simulink model "DLHnguoc_5DOF"  (R2018a)
settings: Solver=VariableStepAuto  StartTime=0.0  StopTime=10.0  RelTol=1e-3
settings Model: Creator=Dell  LastModifiedBy=Nguyen Mai

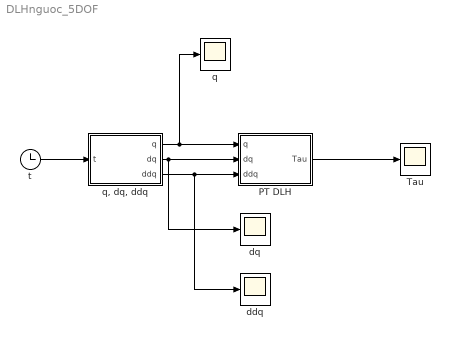
== system DLHnguoc_5DOF ==
  PT DLH : MATLAB Function  TreatAsAtomicUnit=on
  Tau : Scope
  ddq : Scope
  dq : Scope
  q : Scope
  "q, dq, ddq" : MATLAB Function  TreatAsAtomicUnit=on
  t : Clock
  wires:
  "q, dq, ddq"/1(q) -> q/1, PT DLH/1(q)
  t/1 -> "q, dq, ddq"/1(t)
  "q, dq, ddq"/2(dq) -> dq/1, PT DLH/2(dq)
  "q, dq, ddq"/3(ddq) -> ddq/1, PT DLH/3(ddq)
  PT DLH/1(Tau) -> Tau/1

== matlab function DLHnguoc_5DOF/PT DLH ==
  data: q input; Tau output; dq input; ddq input
function Tau=DLHN(q,dq,ddq)
[m1,m2,m3,m4,m5,L1,L2,L3,L4,L5,Lc1,Lc2,Lc3,Lc4,Lc5,g,I1x,I1y,I1z,I2x,I2y,I2z,I3x,I3y,I3z,I4x,I4y,I4z,I5x,I5y,I5z]=parameter ();
ddq=zeros(5,1);
% Khai bao ma tran khoi luong M
M=zeros(5,5);
M(1,1)= m4*L3^2*cos(q(3))^2+m4*cos(q(3))^2*L4^2+I3z+I2y+I1z+(9/4)*m3*L3^2*cos(q(3))^2-(9/4)*L5^2*cos(q(5))^2*cos(q(4))^2*cos(q(3))^2*m5+(9/4)*m2*L2^2-3*m5*cos(q(3))*L5*sin(q(5))*L2+cos(q(3))^2*cos(q(4))^2*I4x+m5*L3^2*cos(q(3))^2+m5*cos(q(3))^2*L4^2-I4y*cos(q(3))^2+cos(q(3))^2*I4z+(1/4)*m4*L4^2+m5*L2^2+I5x*cos(q(3))^2*cos(q(5))^2+I5y*cos(q(4))^2*cos(q(3))^2-I5y*cos(q(3))^2*cos(q(5))^2-I5z*cos(q(4))^2*cos(q(3))^2+(9/4)*L5^2*cos(q(5))^2*m5-2*I5x*cos(q(4))*cos(q(3))*sin(q(3))*cos(q(5))*sin(q(5))+2*I5y*cos(q(4))*cos(q(3))*sin(q(3))*cos(q(5))*sin(q(5))+3*L2*L3*cos(q(3))*m3-(1/4)*L4^2*cos(q(4))^2*cos(q(3))^2*m4+cos(q(3))^2*I3x-I3z*cos(q(3))^2-I5x*cos(q(3))^2-I5x*cos(q(5))^2+I5y*cos(q(5))^2+cos(q(3))^2*I5z-m4*L4*cos(q(4))*sin(q(3))*L2-I4z*cos(q(4))^2*cos(q(3))^2+L2^2*m3+(9/4)*m5*cos(q(3))^2*L5^2+2*m4*cos(q(3))^2*L4*L3+m4*L2^2-I5y*cos(q(4))^2*cos(q(3))^2*cos(q(5))^2-(9/4)*L5^2*cos(q(5))^2*cos(q(3))^2*m5+2*m4*L3*cos(q(3))*L2+2*m4*cos(q(3))*L4*L2+I5x-m4*cos(q(3))*L4^2*sin(q(3))*cos(q(4))+I5x*cos(q(4))^2*cos(q(3))^2*cos(q(5))^2+2*m5*L3*cos(q(3))*L2+2*m5*cos(q(3))*L4*L2+I4y-m4*L3*cos(q(3))*sin(q(3))*cos(q(4))*L4-3*m5*L5*cos(q(5))*cos(q(4))*sin(q(3))*L2+(9/2)*m5*sin(q(3))*cos(q(4))*L5^2*cos(q(5))*cos(q(3))*sin(q(5))-3*m5*sin(q(3))*cos(q(4))*L5*cos(q(5))*L3*cos(q(3))-3*m5*sin(q(3))*cos(q(4))*L5*cos(q(5))*cos(q(3))*L4+2*m5*L3*cos(q(3))^2*L4-3*m5*cos(q(3))^2*L5*sin(q(5))*L3-3*m5*cos(q(3))^2*L5*sin(q(5))*L4;
M(1,2)= 0;
M(1,3)= (1/4)*sin(q(4))*(-9*m5*L5^2*cos(q(5))^2*cos(q(4))*cos(q(3))+9*m5*L5^2*sin(q(5))*cos(q(5))*sin(q(3))+4*I5x*cos(q(5))^2*cos(q(4))*cos(q(3))-4*I5y*cos(q(5))^2*cos(q(4))*cos(q(3))-6*m5*L3*L5*cos(q(5))*sin(q(3))-m4*L4^2*cos(q(4))*cos(q(3))-6*m5*L4*L5*cos(q(5))*sin(q(3))-4*I5x*sin(q(5))*cos(q(5))*sin(q(3))+4*I5y*sin(q(5))*cos(q(5))*sin(q(3))-2*m4*L3*L4*sin(q(3))-2*m4*L4^2*sin(q(3))+4*I4x*cos(q(4))*cos(q(3))-4*I4z*cos(q(4))*cos(q(3))+4*I5y*cos(q(4))*cos(q(3))-4*I5z*cos(q(4))*cos(q(3)));
M(1,4)= (1/4)*m4*L4^2*sin(q(3))-(1/2)*m4*L4^2*cos(q(4))*cos(q(3))-(1/2)*m4*L4*L3*cos(q(4))*cos(q(3))-(1/2)*m4*L4*L2*cos(q(4))+I4y*sin(q(3))-I5x*cos(q(5))^2*sin(q(3))+I5y*cos(q(5))^2*sin(q(3))+(9/4)*m5*L5^2*cos(q(5))^2*sin(q(3))+I5y*sin(q(5))*cos(q(5))*cos(q(4))*cos(q(3))+I5x*sin(q(3))-I5x*sin(q(5))*cos(q(5))*cos(q(4))*cos(q(3))-(3/2)*m5*L5*cos(q(5))*L3*cos(q(4))*cos(q(3))-(3/2)*m5*L5*cos(q(5))*L4*cos(q(4))*cos(q(3))+(9/4)*m5*L5^2*cos(q(5))*sin(q(5))*cos(q(4))*cos(q(3))-(3/2)*m5*L5*cos(q(5))*L2*cos(q(4));
M(1,5)= -(1/4)*sin(q(4))*(-6*m5*L5*L3*sin(q(5))*cos(q(3))-6*m5*L5*L4*sin(q(5))*cos(q(3))-6*m5*L5*L2*sin(q(5))+9*m5*L5^2*cos(q(3))+4*I5z*cos(q(3)));

M(2,1)=0;
M(2,2)=(1/4)*m1;
M(2,3)=0;
M(2,4)=0;
M(2,5)=0;

M(3,1)=(1/4)*sin(q(4))*(-9*m5*L5^2*cos(q(5))^2*cos(q(4))*cos(q(3))+9*m5*L5^2*sin(q(5))*cos(q(5))*sin(q(3))+4*I5x*cos(q(5))^2*cos(q(4))*cos(q(3))-4*I5y*cos(q(5))^2*cos(q(4))*cos(q(3))-6*m5*L3*L5*cos(q(5))*sin(q(3))-m4*L4^2*cos(q(4))*cos(q(3))-6*m5*L4*L5*cos(q(5))*sin(q(3))-4*I5x*sin(q(5))*cos(q(5))*sin(q(3))+4*I5y*sin(q(5))*cos(q(5))*sin(q(3))-2*m4*L3*L4*sin(q(3))-2*m4*L4^2*sin(q(3))+4*I4x*cos(q(4))*cos(q(3))-4*I4z*cos(q(4))*cos(q(3))+4*I5y*cos(q(4))*cos(q(3))-4*I5z*cos(q(4))*cos(q(3)));
M(3,2)=0;
M(3,3)=(9/4)*m3*L3^2+I3y+m4*L3^2+I4z*cos(q(4))^2-I4x*cos(q(4))^2+m4*L4^2+2*m4*L4*L3+(1/4)*m4*cos(q(4))^2*L4^2+I4x+I5y*cos(q(4))^2*cos(q(5))^2-I5x*cos(q(4))^2*cos(q(5))^2+(9/4)*m5*cos(q(4))^2*L5^2*cos(q(5))^2+m5*L3^2+m5*L4^2+2*m5*L3*L4-(9/4)*L5^2*cos(q(5))^2*m5+(9/4)*m5*L5^2-3*L4*L5*sin(q(5))*m5-3*L3*L5*sin(q(5))*m5+I5z*cos(q(4))^2+I5x*cos(q(5))^2-I5y*cos(q(4))^2-I5y*cos(q(5))^2+I5y;
M(3,4)=-(1/4)*sin(q(4))*(-9*L5^2*sin(q(5))*cos(q(5))*m5+6*L3*L5*cos(q(5))*m5+6*L4*L5*cos(q(5))*m5+4*I5x*sin(q(5))*cos(q(5))-4*I5y*sin(q(5))*cos(q(5))+2*m4*L4*L3+2*m4*L4^2);
M(3,5)=(1/4)*cos(q(4))*(-6*L3*L5*sin(q(5))*m5-6*L4*L5*sin(q(5))*m5+9*m5*L5^2+4*I5z);

M(4,1)=(1/4)*m4*L4^2*sin(q(3))-(1/2)*m4*L4^2*cos(q(4))*cos(q(3))-(1/2)*m4*L4*L3*cos(q(4))*cos(q(3))-(1/2)*m4*L4*L2*cos(q(4))+I4y*sin(q(3))-I5x*cos(q(5))^2*sin(q(3))+I5y*cos(q(5))^2*sin(q(3))+(9/4)*m5*L5^2*cos(q(5))^2*sin(q(3))+I5y*sin(q(5))*cos(q(5))*cos(q(4))*cos(q(3))+I5x*sin(q(3))-I5x*sin(q(5))*cos(q(5))*cos(q(4))*cos(q(3))-(3/2)*m5*L5*cos(q(5))*L3*cos(q(4))*cos(q(3))-(3/2)*m5*L5*cos(q(5))*L4*cos(q(4))*cos(q(3))+(9/4)*m5*L5^2*cos(q(5))*sin(q(5))*cos(q(4))*cos(q(3))-(3/2)*m5*L5*cos(q(5))*L2*cos(q(4));
M(4,2)=0;
M(4,3)=-(1/4)*sin(q(4))*(-9*L5^2*sin(q(5))*cos(q(5))*m5+6*L3*L5*cos(q(5))*m5+6*L4*L5*cos(q(5))*m5+4*I5x*sin(q(5))*cos(q(5))-4*I5y*sin(q(5))*cos(q(5))+2*m4*L4*L3+2*m4*L4^2);
M(4,4)=(1/4)*m4*L4^2+I4y+I5y*cos(q(5))^2-I5x*cos(q(5))^2+I5x+(9/4)*L5^2*cos(q(5))^2*m5;
M(4,5)=0;

M(5,1)=-(1/4)*sin(q(4))*(-6*m5*L5*L3*sin(q(5))*cos(q(3))-6*m5*L5*L4*sin(q(5))*cos(q(3))-6*m5*L5*L2*sin(q(5))+9*m5*L5^2*cos(q(3))+4*I5z*cos(q(3)));
M(5,2)=0;
M(5,3)=(1/4)*cos(q(4))*(-6*L3*L5*sin(q(5))*m5-6*L4*L5*sin(q(5))*m5+9*m5*L5^2+4*I5z);
M(5,4)=0;
M(5,5)=(9/4)*m5*L5^2+I5z;

% Khai bao ma tran Coriolis C
%h=-m2*L1*Lc2*sin(q(2));
Co=zeros(5,5);
Co(1,1)=-2*sin(q(4))*dq(4)*cos(q(3))^2*cos(q(4))*I4x-2*sin(q(4))*dq(4)*I5y*cos(q(4))*cos(q(3))^2+2*sin(q(4))*dq(4)*I5z*cos(q(4))*cos(q(3))^2+2*sin(q(4))*dq(4)*I4z*cos(q(4))*cos(q(3))^2-2*dq(3)*m4*cos(q(3))^2*L4^2*cos(q(4))-2*dq(3)*m4*sin(q(3))*L4*L2-2*dq(3)*m4*cos(q(3))*L4^2*sin(q(3))-2*dq(3)*m4*L3*sin(q(3))*L2-2*dq(3)*m5*L3*sin(q(3))*L2-2*dq(3)*m5*sin(q(3))*L4*L2-2*dq(3)*m4*L3^2*cos(q(3))*sin(q(3))-(9/2)*dq(3)*m3*L3^2*cos(q(3))*sin(q(3))-2*dq(3)*cos(q(3))*cos(q(4))^2*I4x*sin(q(3))-2*dq(3)*m5*L3^2*cos(q(3))*sin(q(3))-2*dq(3)*m5*cos(q(3))*L4^2*sin(q(3))-2*dq(3)*I5x*cos(q(3))*cos(q(5))^2*sin(q(3))-2*dq(3)*I5y*cos(q(4))^2*cos(q(3))*sin(q(3))+2*dq(3)*I5y*cos(q(3))*cos(q(5))^2*sin(q(3))+2*dq(3)*I5z*cos(q(4))^2*cos(q(3))*sin(q(3))-3*dq(3)*L2*L3*sin(q(3))*m3+2*dq(3)*I4z*cos(q(4))^2*cos(q(3))*sin(q(3))-(9/2)*dq(3)*m5*cos(q(3))*L5^2*sin(q(3))+2*dq(5)*I5x*cos(q(4))*cos(q(3))*sin(q(3))-2*dq(5)*I5y*cos(q(4))*cos(q(3))*sin(q(3))-2*dq(5)*I5x*cos(q(3))^2*cos(q(5))*sin(q(5))+2*dq(5)*I5y*cos(q(3))^2*cos(q(5))*sin(q(5))-(9/2)*L5^2*cos(q(4))*sin(q(5))*cos(q(5))*dq(3)*m5-(9/2)*L5^2*sin(q(5))*cos(q(5))*dq(5)*m5+2*I5x*cos(q(4))*sin(q(5))*cos(q(5))*dq(3)-2*I5y*cos(q(4))*sin(q(5))*cos(q(5))*dq(3)+L3*L4*cos(q(4))*dq(3)*m4+2*dq(3)*I4y*cos(q(3))*sin(q(3))-2*dq(3)*cos(q(3))*I3x*sin(q(3))+2*dq(3)*I3z*cos(q(3))*sin(q(3))+2*dq(3)*I5x*cos(q(3))*sin(q(3))-2*dq(3)*cos(q(3))*I5z*sin(q(3))-2*dq(3)*cos(q(3))*I4z*sin(q(3))+3*sin(q(4))*dq(4)*m5*sin(q(3))*L5*cos(q(5))*cos(q(3))*L4+3*sin(q(4))*dq(4)*m5*sin(q(3))*L5*cos(q(5))*L3*cos(q(3))-(9/2)*sin(q(4))*dq(4)*m5*sin(q(3))*L5^2*cos(q(5))*cos(q(3))*sin(q(5))+3*dq(5)*m5*sin(q(3))*cos(q(4))*L5*sin(q(5))*cos(q(3))*L4+3*dq(5)*m5*sin(q(3))*cos(q(4))*L5*sin(q(5))*L3*cos(q(3))+(9/2)*sin(q(4))*dq(4)*L5^2*cos(q(5))^2*cos(q(4))*cos(q(3))^2*m5+2*sin(q(4))*dq(4)*I5x*cos(q(3))*sin(q(3))*cos(q(5))*sin(q(5))-2*sin(q(4))*dq(4)*I5y*cos(q(3))*sin(q(3))*cos(q(5))*sin(q(5))+sin(q(4))*dq(4)*m4*cos(q(3))*L4*L3*sin(q(3))+3*sin(q(4))*dq(4)*m5*L5*cos(q(5))*sin(q(3))*L2+9*dq(3)*m5*cos(q(3))^2*cos(q(4))*L5^2*cos(q(5))*sin(q(5))-6*dq(3)*m5*cos(q(3))^2*cos(q(4))*L5*cos(q(5))*L3-6*dq(3)*m5*cos(q(3))^2*cos(q(4))*L5*cos(q(5))*L4-3*dq(3)*m5*L5*cos(q(5))*cos(q(4))*cos(q(3))*L2+6*dq(3)*m5*cos(q(3))*L5*sin(q(5))*L3*sin(q(3))+6*dq(3)*m5*cos(q(3))*L5*sin(q(5))*L4*sin(q(3))+(9/2)*dq(3)*L5^2*cos(q(5))^2*cos(q(4))^2*cos(q(3))*m5*sin(q(3))+(9/2)*dq(5)*L5^2*cos(q(5))*cos(q(4))^2*cos(q(3))^2*m5*sin(q(5))+9*dq(5)*m5*sin(q(3))*cos(q(4))*L5^2*cos(q(5))^2*cos(q(3))+3*dq(5)*m5*L5*sin(q(5))*cos(q(4))*sin(q(3))*L2+(1/2)*sin(q(4))*dq(4)*m4*cos(q(3))^2*L4^2*cos(q(4))+sin(q(4))*dq(4)*m4*sin(q(3))*L4*L2+2*sin(q(4))*dq(4)*I5y*cos(q(4))*cos(q(3))^2*cos(q(5))^2+sin(q(4))*dq(4)*m4*cos(q(3))*L4^2*sin(q(3))-2*sin(q(4))*dq(4)*I5x*cos(q(4))*cos(q(3))^2*cos(q(5))^2-4*dq(3)*m4*cos(q(3))*L4*L3*sin(q(3))-2*dq(3)*I5x*cos(q(4))^2*cos(q(3))*cos(q(5))^2*sin(q(3))-4*dq(3)*m5*L3*cos(q(3))*L4*sin(q(3))+3*dq(3)*m5*sin(q(3))*L5*sin(q(5))*L2+(1/2)*dq(3)*L4^2*cos(q(4))^2*cos(q(3))*m4*sin(q(3))-dq(3)*m4*L4*cos(q(4))*cos(q(3))*L2+2*dq(3)*I5y*cos(q(4))^2*cos(q(3))*cos(q(5))^2*sin(q(3))+(9/2)*dq(3)*L5^2*cos(q(5))^2*cos(q(3))*m5*sin(q(3))-2*dq(3)*m4*L3*cos(q(3))^2*cos(q(4))*L4-4*dq(3)*I5x*cos(q(4))*cos(q(3))^2*cos(q(5))*sin(q(5))+4*dq(3)*I5y*cos(q(4))*cos(q(3))^2*cos(q(5))*sin(q(5))-(9/2)*dq(5)*m5*sin(q(3))*cos(q(4))*L5^2*cos(q(3))-2*dq(5)*I5x*cos(q(4))^2*cos(q(3))^2*cos(q(5))*sin(q(5))+2*dq(5)*I5y*cos(q(4))^2*cos(q(3))^2*cos(q(5))*sin(q(5))+(9/2)*dq(5)*L5^2*cos(q(5))*cos(q(3))^2*m5*sin(q(5))-4*dq(5)*I5x*cos(q(4))*cos(q(3))*sin(q(3))*cos(q(5))^2+4*dq(5)*I5y*cos(q(4))*cos(q(3))*sin(q(3))*cos(q(5))^2-3*dq(5)*m5*cos(q(3))^2*L5*cos(q(5))*L3-3*dq(5)*m5*cos(q(3))^2*L5*cos(q(5))*L4-3*dq(5)*m5*cos(q(3))*L5*cos(q(5))*L2+3*L3*L5*cos(q(4))*cos(q(5))*dq(3)*m5+3*L4*L5*cos(q(4))*cos(q(5))*dq(3)*m5+2*I5x*sin(q(5))*cos(q(5))*dq(5)-2*I5y*sin(q(5))*cos(q(5))*dq(5)+L4^2*cos(q(4))*dq(3)*m4;
Co(1,2)=0;
Co(1,3)=-sin(q(4))*dq(3)*I5x*cos(q(5))^2*cos(q(4))*sin(q(3))+sin(q(4))*dq(3)*I5y*cos(q(5))^2*cos(q(4))*sin(q(3))+(1/4)*sin(q(4))*dq(3)*L4^2*cos(q(4))*sin(q(3))*m4-sin(q(4))*dq(3)*I5x*cos(q(5))*cos(q(3))*sin(q(5))+sin(q(4))*dq(3)*I5y*cos(q(5))*cos(q(3))*sin(q(5))-(1/2)*sin(q(4))*dq(3)*m4*L4*L3*cos(q(3))-(9/2)*dq(4)*L5^2*cos(q(4))^2*cos(q(5))^2*cos(q(3))*m5-dq(4)*I5x*cos(q(4))*sin(q(5))*cos(q(5))*sin(q(3))+dq(4)*I5y*cos(q(4))*sin(q(5))*cos(q(5))*sin(q(3))-(1/2)*dq(4)*L3*L4*cos(q(4))*sin(q(3))*m4+(9/2)*L5^2*cos(q(5))^2*sin(q(3))*sin(q(4))*dq(5)*m5-(1/2)*sin(q(4))*dq(3)*m4*L4^2*cos(q(3))-sin(q(4))*dq(3)*I4x*cos(q(4))*sin(q(3))+sin(q(4))*dq(3)*I4z*cos(q(4))*sin(q(3))-sin(q(4))*dq(3)*I5y*cos(q(4))*sin(q(3))+sin(q(4))*dq(3)*I5z*cos(q(4))*sin(q(3))+(9/4)*dq(4)*L5^2*cos(q(5))^2*cos(q(3))*m5+2*dq(4)*I5x*cos(q(4))^2*cos(q(5))^2*cos(q(3))-2*dq(4)*I5y*cos(q(4))^2*cos(q(5))^2*cos(q(3))-(1/2)*dq(4)*L4^2*cos(q(4))^2*cos(q(3))*m4-(1/2)*dq(4)*L4^2*cos(q(4))*sin(q(3))*m4-2*I5x*cos(q(5))^2*sin(q(3))*sin(q(4))*dq(5)+2*I5y*cos(q(5))^2*sin(q(3))*sin(q(4))*dq(5)-(9/4)*L5^2*sin(q(3))*sin(q(4))*dq(5)*m5-dq(4)*I4x*cos(q(3))+dq(4)*I4z*cos(q(3))-dq(4)*I5y*cos(q(3))+dq(4)*I5z*cos(q(3))-I5y*sin(q(3))*sin(q(4))*dq(5)+2*dq(4)*I4x*cos(q(4))^2*cos(q(3))-2*dq(4)*I4z*cos(q(4))^2*cos(q(3))+2*dq(4)*I5y*cos(q(4))^2*cos(q(3))-2*dq(4)*I5z*cos(q(4))^2*cos(q(3))-dq(4)*I5x*cos(q(5))^2*cos(q(3))+dq(4)*I5y*cos(q(5))^2*cos(q(3))+(1/4)*dq(4)*m4*L4^2*cos(q(3))+I5x*sin(q(3))*sin(q(4))*dq(5)+(9/2)*L5^2*cos(q(4))*sin(q(5))*cos(q(5))*cos(q(3))*sin(q(4))*dq(5)*m5-2*I5x*cos(q(4))*sin(q(5))*cos(q(5))*cos(q(3))*sin(q(4))*dq(5)+2*I5y*cos(q(4))*sin(q(5))*cos(q(5))*cos(q(3))*sin(q(4))*dq(5)+(3/2)*L3*L5*sin(q(5))*sin(q(3))*sin(q(4))*dq(5)*m5+(3/2)*L4*L5*sin(q(5))*sin(q(3))*sin(q(4))*dq(5)*m5+(9/4)*sin(q(4))*dq(3)*m5*L5^2*cos(q(5))^2*cos(q(4))*sin(q(3))+(9/4)*sin(q(4))*dq(3)*m5*L5^2*cos(q(5))*sin(q(5))*cos(q(3))-(3/2)*sin(q(4))*dq(3)*m5*L5*cos(q(5))*L3*cos(q(3))-(3/2)*sin(q(4))*dq(3)*m5*L5*cos(q(5))*L4*cos(q(3))+(9/4)*dq(4)*L5^2*cos(q(4))*sin(q(5))*cos(q(5))*sin(q(3))*m5-(3/2)*dq(4)*L3*L5*cos(q(4))*cos(q(5))*sin(q(3))*m5-(3/2)*dq(4)*L4*L5*cos(q(4))*cos(q(5))*sin(q(3))*m5;
Co(1,4)=dq(3)*I4y*cos(q(3))+dq(3)*I5x*cos(q(3))+(1/2)*dq(3)*L4^2*cos(q(4))*sin(q(3))*m4+(9/4)*dq(3)*L5^2*cos(q(5))^2*cos(q(3))*m5-(9/4)*dq(5)*L5^2*cos(q(4))*cos(q(3))*m5-2*dq(5)*I5x*cos(q(5))^2*cos(q(4))*cos(q(3))+2*dq(5)*I5y*cos(q(5))^2*cos(q(4))*cos(q(3))+2*dq(5)*I5x*sin(q(5))*cos(q(5))*sin(q(3))-2*dq(5)*I5y*sin(q(5))*cos(q(5))*sin(q(3))+(1/2)*L4^2*cos(q(3))*sin(q(4))*dq(4)*m4+(1/2)*L2*L4*sin(q(4))*dq(4)*m4+(1/2)*dq(3)*L3*L4*cos(q(4))*sin(q(3))*m4-dq(3)*I5y*cos(q(4))*sin(q(5))*cos(q(5))*sin(q(3))+dq(3)*I5x*cos(q(4))*sin(q(5))*cos(q(5))*sin(q(3))+(9/2)*dq(5)*m5*L5^2*cos(q(5))^2*cos(q(4))*cos(q(3))-(9/2)*dq(5)*m5*L5^2*sin(q(5))*cos(q(5))*sin(q(3))+(3/2)*dq(5)*L2*L5*cos(q(4))*sin(q(5))*m5+I5x*sin(q(5))*cos(q(5))*cos(q(3))*sin(q(4))*dq(4)-I5y*sin(q(5))*cos(q(5))*cos(q(3))*sin(q(4))*dq(4)+(3/2)*L2*L5*cos(q(5))*sin(q(4))*dq(4)*m5+(1/2)*L3*L4*cos(q(3))*sin(q(4))*dq(4)*m4+(1/4)*dq(3)*m4*L4^2*cos(q(3))-dq(3)*I5x*cos(q(5))^2*cos(q(3))+dq(3)*I5y*cos(q(5))^2*cos(q(3))+dq(5)*I5x*cos(q(4))*cos(q(3))-dq(5)*I5y*cos(q(4))*cos(q(3))+(3/2)*dq(3)*L4*L5*cos(q(4))*cos(q(5))*sin(q(3))*m5-(9/4)*dq(3)*L5^2*cos(q(4))*sin(q(5))*cos(q(5))*sin(q(3))*m5+(3/2)*dq(5)*L3*L5*cos(q(4))*sin(q(5))*cos(q(3))*m5+(3/2)*dq(5)*L4*L5*cos(q(4))*sin(q(5))*cos(q(3))*m5-(9/4)*L5^2*sin(q(5))*cos(q(5))*cos(q(3))*sin(q(4))*dq(4)*m5+(3/2)*L3*L5*cos(q(5))*cos(q(3))*sin(q(4))*dq(4)*m5+(3/2)*L4*L5*cos(q(5))*cos(q(3))*sin(q(4))*dq(4)*m5+(3/2)*dq(3)*L3*L5*cos(q(4))*cos(q(5))*sin(q(3))*m5;
Co(1,5)=(3/2)*L3*L5*cos(q(4))*sin(q(5))*cos(q(3))*dq(4)*m5-(3/2)*L3*L5*sin(q(5))*sin(q(3))*sin(q(4))*dq(3)*m5+(3/2)*L3*L5*cos(q(5))*cos(q(3))*sin(q(4))*dq(5)*m5+(3/2)*L4*L5*cos(q(4))*sin(q(5))*cos(q(3))*dq(4)*m5-(3/2)*L4*L5*sin(q(5))*sin(q(3))*sin(q(4))*dq(3)*m5+(3/2)*L4*L5*cos(q(5))*cos(q(3))*sin(q(4))*dq(5)*m5+(3/2)*L2*L5*cos(q(4))*sin(q(5))*dq(4)*m5+(3/2)*L2*L5*cos(q(5))*sin(q(4))*dq(5)*m5-(9/4)*L5^2*cos(q(4))*cos(q(3))*dq(4)*m5+(9/4)*L5^2*sin(q(3))*sin(q(4))*dq(3)*m5-I5z*cos(q(4))*cos(q(3))*dq(4)+I5z*sin(q(3))*sin(q(4))*dq(3);

Co(2,1)=0;
Co(2,2)=0;
Co(2,3)=0;
Co(2,4)=0;
Co(2,5)=0;

Co(3,1)=-(1/2)*sin(q(4))*dq(3)*I5x*cos(q(5))^2*cos(q(4))*sin(q(3))+(1/2)*sin(q(4))*dq(3)*I5y*cos(q(5))^2*cos(q(4))*sin(q(3))+(1/8)*sin(q(4))*dq(3)*L4^2*cos(q(4))*sin(q(3))*m4-(1/2)*sin(q(4))*dq(3)*I5x*cos(q(5))*cos(q(3))*sin(q(5))+(1/2)*sin(q(4))*dq(3)*I5y*cos(q(5))*cos(q(3))*sin(q(5))-(1/4)*sin(q(4))*dq(3)*m4*L4*L3*cos(q(3))-(9/2)*dq(4)*L5^2*cos(q(4))^2*cos(q(5))^2*cos(q(3))*m5-(3/2)*dq(4)*I5x*cos(q(4))*sin(q(5))*cos(q(5))*sin(q(3))+(3/2)*dq(4)*I5y*cos(q(4))*sin(q(5))*cos(q(5))*sin(q(3))-(3/4)*dq(4)*L3*L4*cos(q(4))*sin(q(3))*m4+(9/2)*L5^2*cos(q(5))^2*sin(q(3))*sin(q(4))*dq(5)*m5-(1/4)*sin(q(4))*dq(3)*m4*L4^2*cos(q(3))-(1/2)*sin(q(4))*dq(3)*I4x*cos(q(4))*sin(q(3))+(1/2)*sin(q(4))*dq(3)*I4z*cos(q(4))*sin(q(3))-(1/2)*sin(q(4))*dq(3)*I5y*cos(q(4))*sin(q(3))+(1/2)*sin(q(4))*dq(3)*I5z*cos(q(4))*sin(q(3))+(9/8)*dq(4)*L5^2*cos(q(5))^2*cos(q(3))*m5+2*dq(4)*I5x*cos(q(4))^2*cos(q(5))^2*cos(q(3))-2*dq(4)*I5y*cos(q(4))^2*cos(q(5))^2*cos(q(3))-(1/2)*dq(4)*L4^2*cos(q(4))^2*cos(q(3))*m4-(3/4)*dq(4)*L4^2*cos(q(4))*sin(q(3))*m4-2*I5x*cos(q(5))^2*sin(q(3))*sin(q(4))*dq(5)+2*I5y*cos(q(5))^2*sin(q(3))*sin(q(4))*dq(5)-(27/8)*L5^2*sin(q(3))*sin(q(4))*dq(5)*m5-dq(4)*I4x*cos(q(3))+dq(4)*I4z*cos(q(3))-dq(4)*I5y*cos(q(3))+dq(4)*I5z*cos(q(3))-(1/2)*dq(4)*I4y*cos(q(3))-I5y*sin(q(3))*sin(q(4))*dq(5)+2*dq(4)*I4x*cos(q(4))^2*cos(q(3))-2*dq(4)*I4z*cos(q(4))^2*cos(q(3))+2*dq(4)*I5y*cos(q(4))^2*cos(q(3))-2*dq(4)*I5z*cos(q(4))^2*cos(q(3))-(1/2)*dq(4)*I5x*cos(q(5))^2*cos(q(3))+(1/2)*dq(4)*I5y*cos(q(5))^2*cos(q(3))+(1/8)*dq(4)*m4*L4^2*cos(q(3))+I5x*sin(q(3))*sin(q(4))*dq(5)+(9/4)*dq(1)*m5*cos(q(3))*L5^2*sin(q(3))+dq(1)*m4*cos(q(3))^2*L4^2*cos(q(4))-(1/2)*dq(1)*m4*L3*cos(q(4))*L4-dq(1)*I5x*sin(q(5))*cos(q(5))*cos(q(4))+dq(1)*I5y*sin(q(5))*cos(q(5))*cos(q(4))+dq(1)*m4*L3*sin(q(3))*L2+dq(1)*m4*sin(q(3))*L4*L2+dq(1)*m5*L3*sin(q(3))*L2+dq(1)*m5*sin(q(3))*L4*L2+dq(1)*m4*L3^2*cos(q(3))*sin(q(3))+dq(1)*m4*cos(q(3))*L4^2*sin(q(3))+(9/4)*dq(1)*m3*L3^2*cos(q(3))*sin(q(3))+dq(1)*cos(q(3))*cos(q(4))^2*I4x*sin(q(3))+dq(1)*m5*L3^2*cos(q(3))*sin(q(3))+dq(1)*m5*cos(q(3))*L4^2*sin(q(3))+dq(1)*I5x*cos(q(3))*cos(q(5))^2*sin(q(3))+dq(1)*I5y*cos(q(4))^2*cos(q(3))*sin(q(3))-dq(1)*I5y*cos(q(3))*cos(q(5))^2*sin(q(3))-dq(1)*I5z*cos(q(4))^2*cos(q(3))*sin(q(3))+(3/2)*dq(1)*L2*L3*sin(q(3))*m3-dq(1)*I4z*cos(q(4))^2*cos(q(3))*sin(q(3))+(9/2)*L5^2*cos(q(4))*sin(q(5))*cos(q(5))*cos(q(3))*sin(q(4))*dq(5)*m5+3*dq(1)*m5*cos(q(3))^2*cos(q(4))*L5*cos(q(5))*L3+3*dq(1)*m5*cos(q(3))^2*cos(q(4))*L5*cos(q(5))*L4+(3/2)*dq(1)*m5*L5*cos(q(5))*cos(q(4))*cos(q(3))*L2-3*dq(1)*m5*cos(q(3))*L5*sin(q(5))*L3*sin(q(3))-3*dq(1)*m5*cos(q(3))*L5*sin(q(5))*L4*sin(q(3))-(9/4)*dq(1)*L5^2*cos(q(5))^2*cos(q(4))^2*cos(q(3))*m5*sin(q(3))-(9/2)*dq(1)*m5*cos(q(3))^2*cos(q(4))*L5^2*cos(q(5))*sin(q(5))-2*I5x*cos(q(4))*sin(q(5))*cos(q(5))*cos(q(3))*sin(q(4))*dq(5)+2*I5y*cos(q(4))*sin(q(5))*cos(q(5))*cos(q(3))*sin(q(4))*dq(5)+(9/4)*L3*L5*sin(q(5))*sin(q(3))*sin(q(4))*dq(5)*m5+(9/4)*L4*L5*sin(q(5))*sin(q(3))*sin(q(4))*dq(5)*m5+(9/8)*sin(q(4))*dq(3)*m5*L5^2*cos(q(5))^2*cos(q(4))*sin(q(3))+(9/8)*sin(q(4))*dq(3)*m5*L5^2*cos(q(5))*sin(q(5))*cos(q(3))-(3/4)*sin(q(4))*dq(3)*m5*L5*cos(q(5))*L3*cos(q(3))-(3/4)*sin(q(4))*dq(3)*m5*L5*cos(q(5))*L4*cos(q(3))+(27/8)*dq(4)*L5^2*cos(q(4))*sin(q(5))*cos(q(5))*sin(q(3))*m5-(9/4)*dq(4)*L3*L5*cos(q(4))*cos(q(5))*sin(q(3))*m5-(9/4)*dq(4)*L4*L5*cos(q(4))*cos(q(5))*sin(q(3))*m5-(1/2)*dq(4)*I5x*cos(q(3))+2*dq(1)*I5x*cos(q(4))*cos(q(3))^2*cos(q(5))*sin(q(5))-2*dq(1)*I5y*cos(q(4))*cos(q(3))^2*cos(q(5))*sin(q(5))+(9/4)*dq(1)*m5*cos(q(4))*L5^2*cos(q(5))*sin(q(5))-(3/2)*dq(1)*m5*cos(q(4))*L5*cos(q(5))*L3-(3/2)*dq(1)*m5*cos(q(4))*L5*cos(q(5))*L4+dq(1)*I5x*cos(q(4))^2*cos(q(3))*cos(q(5))^2*sin(q(3))+2*dq(1)*m5*L3*cos(q(3))*L4*sin(q(3))-(3/2)*dq(1)*m5*sin(q(3))*L5*sin(q(5))*L2-(1/4)*dq(1)*L4^2*cos(q(4))^2*cos(q(3))*m4*sin(q(3))+(1/2)*dq(1)*m4*L4*cos(q(4))*cos(q(3))*L2+2*dq(1)*m4*cos(q(3))*L4*L3*sin(q(3))-dq(1)*I5y*cos(q(4))^2*cos(q(3))*cos(q(5))^2*sin(q(3))-(9/4)*dq(1)*L5^2*cos(q(5))^2*cos(q(3))*m5*sin(q(3))+dq(1)*m4*L3*cos(q(3))^2*cos(q(4))*L4-(1/2)*dq(1)*m4*L4^2*cos(q(4))-dq(1)*I4y*cos(q(3))*sin(q(3))+dq(1)*cos(q(3))*I3x*sin(q(3))-dq(1)*I3z*cos(q(3))*sin(q(3))-dq(1)*I5x*cos(q(3))*sin(q(3))+dq(1)*cos(q(3))*I5z*sin(q(3))+dq(1)*cos(q(3))*I4z*sin(q(3))-(1/2)*I5z*sin(q(3))*sin(q(4))*dq(5);
Co(3,2)=0;
Co(3,3)=(1/2)*I5x*sin(q(5))*cos(q(5))*cos(q(3))*sin(q(4))*dq(1)-(1/2)*I5y*sin(q(5))*cos(q(5))*cos(q(3))*sin(q(4))*dq(1)+(1/4)*L3*L4*cos(q(3))*sin(q(4))*dq(1)*m4+2*I4x*cos(q(4))*sin(q(4))*dq(4)-2*I4z*cos(q(4))*sin(q(4))*dq(4)+2*I5y*cos(q(4))*sin(q(4))*dq(4)-2*I5z*cos(q(4))*sin(q(4))*dq(4)+(1/2)*sin(q(4))*dq(1)*I5x*cos(q(5))^2*cos(q(4))*sin(q(3))-(1/2)*sin(q(4))*dq(1)*I5y*cos(q(5))^2*cos(q(4))*sin(q(3))-(1/8)*sin(q(4))*dq(1)*L4^2*cos(q(4))*sin(q(3))*m4-(9/2)*L5^2*cos(q(4))^2*sin(q(5))*cos(q(5))*dq(5)*m5-(9/2)*L5^2*cos(q(4))*cos(q(5))^2*sin(q(4))*dq(4)*m5-(9/8)*L5^2*sin(q(5))*cos(q(5))*cos(q(3))*sin(q(4))*dq(1)*m5+(9/2)*L5^2*sin(q(5))*cos(q(5))*dq(5)*m5+(1/4)*L4^2*cos(q(3))*sin(q(4))*dq(1)*m4-(9/8)*sin(q(4))*dq(1)*m5*L5^2*cos(q(5))^2*cos(q(4))*sin(q(3))+(1/2)*sin(q(4))*dq(1)*I4x*cos(q(4))*sin(q(3))-(1/2)*sin(q(4))*dq(1)*I4z*cos(q(4))*sin(q(3))+(1/2)*sin(q(4))*dq(1)*I5y*cos(q(4))*sin(q(3))-(1/2)*sin(q(4))*dq(1)*I5z*cos(q(4))*sin(q(3))+2*I5x*cos(q(4))^2*sin(q(5))*cos(q(5))*dq(5)-2*I5y*cos(q(4))^2*sin(q(5))*cos(q(5))*dq(5)-3*L3*L5*cos(q(5))*dq(5)*m5-3*L4*L5*cos(q(5))*dq(5)*m5+2*I5x*cos(q(4))*cos(q(5))^2*sin(q(4))*dq(4)-2*I5y*cos(q(4))*cos(q(5))^2*sin(q(4))*dq(4)-(1/2)*L4^2*cos(q(4))*sin(q(4))*dq(4)*m4+(3/4)*L3*L5*cos(q(5))*cos(q(3))*sin(q(4))*dq(1)*m5+(3/4)*L4*L5*cos(q(5))*cos(q(3))*sin(q(4))*dq(1)*m5-2*I5x*sin(q(5))*cos(q(5))*dq(5)+2*I5y*sin(q(5))*cos(q(5))*dq(5);
Co(3,4)=-(1/4)*dq(1)*L3*L4*cos(q(4))*sin(q(3))*m4+(1/2)*dq(1)*I5y*cos(q(4))*sin(q(5))*cos(q(5))*sin(q(3))-(1/2)*dq(1)*I5x*cos(q(4))*sin(q(5))*cos(q(5))*sin(q(3))+(9/4)*L5^2*cos(q(4))*sin(q(5))*cos(q(5))*dq(4)*m5-(3/2)*L3*L5*cos(q(4))*cos(q(5))*dq(4)*m5-(3/2)*L4*L5*cos(q(4))*cos(q(5))*dq(4)*m5+(3/2)*L3*L5*sin(q(5))*sin(q(4))*dq(5)*m5+(3/2)*L4*L5*sin(q(5))*sin(q(4))*dq(5)*m5+(1/2)*dq(1)*I5x*cos(q(5))^2*cos(q(3))-(1/2)*dq(1)*I5y*cos(q(5))^2*cos(q(3))-(1/2)*L4^2*cos(q(4))*dq(4)*m4-2*I5x*cos(q(5))^2*sin(q(4))*dq(5)+2*I5y*cos(q(5))^2*sin(q(4))*dq(5)-(9/4)*L5^2*sin(q(4))*dq(5)*m5-(1/8)*dq(1)*m4*L4^2*cos(q(3))-(1/2)*dq(1)*I5x*cos(q(3))+I5x*sin(q(4))*dq(5)-I5y*sin(q(4))*dq(5)-(1/2)*dq(1)*I4y*cos(q(3))-(3/4)*dq(1)*L4*L5*cos(q(4))*cos(q(5))*sin(q(3))*m5+(9/8)*dq(1)*L5^2*cos(q(4))*sin(q(5))*cos(q(5))*sin(q(3))*m5-(3/4)*dq(1)*L3*L5*cos(q(4))*cos(q(5))*sin(q(3))*m5-(1/4)*dq(1)*L4^2*cos(q(4))*sin(q(3))*m4-(9/8)*dq(1)*L5^2*cos(q(5))^2*cos(q(3))*m5-I5x*cos(q(4))*sin(q(5))*cos(q(5))*dq(4)+I5y*cos(q(4))*sin(q(5))*cos(q(5))*dq(4)-(1/2)*L3*L4*cos(q(4))*dq(4)*m4+(9/2)*L5^2*cos(q(5))^2*sin(q(4))*dq(5)*m5;
Co(3,5)=(3/4)*L3*L5*sin(q(5))*sin(q(3))*sin(q(4))*dq(1)*m5+(3/4)*L4*L5*sin(q(5))*sin(q(3))*sin(q(4))*dq(1)*m5-(3/2)*cos(q(4))*L5*cos(q(5))*m5*dq(5)*L3+(3/2)*L3*L5*sin(q(5))*sin(q(4))*dq(4)*m5-(3/2)*cos(q(4))*L5*cos(q(5))*m5*dq(5)*L4+(3/2)*L4*L5*sin(q(5))*sin(q(4))*dq(4)*m5-(9/8)*L5^2*sin(q(3))*sin(q(4))*dq(1)*m5-(9/4)*L5^2*sin(q(4))*dq(4)*m5-(1/2)*I5z*sin(q(3))*sin(q(4))*dq(1)-I5z*sin(q(4))*dq(4);

Co(4,1)=sin(q(4))*dq(1)*cos(q(3))^2*cos(q(4))*I4x+sin(q(4))*dq(1)*I5y*cos(q(4))*cos(q(3))^2-sin(q(4))*dq(1)*I5z*cos(q(4))*cos(q(3))^2-sin(q(4))*dq(1)*I4z*cos(q(4))*cos(q(3))^2-dq(3)*I5x*cos(q(4))^2*cos(q(5))^2*cos(q(3))+dq(3)*I5y*cos(q(4))^2*cos(q(5))^2*cos(q(3))+(1/4)*dq(3)*L4^2*cos(q(4))^2*cos(q(3))*m4-dq(3)*I4x*cos(q(4))^2*cos(q(3))+dq(3)*I4z*cos(q(4))^2*cos(q(3))-dq(3)*I5y*cos(q(4))^2*cos(q(3))+dq(3)*I5z*cos(q(4))^2*cos(q(3))+(1/2)*I5z*cos(q(4))*cos(q(3))*dq(5)-(1/4)*sin(q(4))*dq(1)*m4*cos(q(3))^2*L4^2*cos(q(4))-(1/2)*sin(q(4))*dq(1)*m4*sin(q(3))*L4*L2-sin(q(4))*dq(1)*I5y*cos(q(4))*cos(q(3))^2*cos(q(5))^2-(1/2)*sin(q(4))*dq(1)*m4*cos(q(3))*L4^2*sin(q(3))+sin(q(4))*dq(1)*I5x*cos(q(4))*cos(q(3))^2*cos(q(5))^2+(9/4)*dq(3)*L5^2*cos(q(4))^2*cos(q(5))^2*cos(q(3))*m5+(9/4)*sin(q(4))*dq(1)*m5*sin(q(3))*L5^2*cos(q(5))*cos(q(3))*sin(q(5))-(3/2)*sin(q(4))*dq(1)*m5*sin(q(3))*L5*cos(q(5))*L3*cos(q(3))-(3/2)*sin(q(4))*dq(1)*m5*sin(q(3))*L5*cos(q(5))*cos(q(3))*L4-(9/4)*sin(q(4))*dq(1)*L5^2*cos(q(5))^2*cos(q(4))*cos(q(3))^2*m5-sin(q(4))*dq(1)*I5x*cos(q(3))*sin(q(3))*cos(q(5))*sin(q(5))+sin(q(4))*dq(1)*I5y*cos(q(3))*sin(q(3))*cos(q(5))*sin(q(5))-(1/2)*sin(q(4))*dq(1)*m4*cos(q(3))*L4*L3*sin(q(3))-(3/2)*sin(q(4))*dq(1)*m5*L5*cos(q(5))*sin(q(3))*L2+(1/2)*dq(3)*I5y*cos(q(3))+dq(3)*I4y*cos(q(3))+dq(3)*I5x*cos(q(3))+(1/2)*dq(3)*I4x*cos(q(3))-(1/2)*dq(3)*I4z*cos(q(3))-(1/2)*dq(3)*I5z*cos(q(3))+(3/4)*dq(3)*L4^2*cos(q(4))*sin(q(3))*m4+(9/8)*dq(3)*L5^2*cos(q(5))^2*cos(q(3))*m5-(9/8)*dq(5)*L5^2*cos(q(4))*cos(q(3))*m5-2*dq(5)*I5x*cos(q(5))^2*cos(q(4))*cos(q(3))+2*dq(5)*I5y*cos(q(5))^2*cos(q(4))*cos(q(3))+2*dq(5)*I5x*sin(q(5))*cos(q(5))*sin(q(3))-2*dq(5)*I5y*sin(q(5))*cos(q(5))*sin(q(3))+(1/4)*L4^2*cos(q(3))*sin(q(4))*dq(4)*m4+(1/4)*L2*L4*sin(q(4))*dq(4)*m4+(3/4)*dq(3)*L3*L4*cos(q(4))*sin(q(3))*m4-(3/2)*dq(3)*I5y*cos(q(4))*sin(q(5))*cos(q(5))*sin(q(3))+(3/2)*dq(3)*I5x*cos(q(4))*sin(q(5))*cos(q(5))*sin(q(3))+(9/2)*dq(5)*m5*L5^2*cos(q(5))^2*cos(q(4))*cos(q(3))-(9/2)*dq(5)*m5*L5^2*sin(q(5))*cos(q(5))*sin(q(3))+(3/4)*dq(5)*L2*L5*cos(q(4))*sin(q(5))*m5+(1/2)*I5x*sin(q(5))*cos(q(5))*cos(q(3))*sin(q(4))*dq(4)-(1/2)*I5y*sin(q(5))*cos(q(5))*cos(q(3))*sin(q(4))*dq(4)+(3/4)*L2*L5*cos(q(5))*sin(q(4))*dq(4)*m5+(1/4)*L3*L4*cos(q(3))*sin(q(4))*dq(4)*m4+(1/8)*dq(3)*m4*L4^2*cos(q(3))-(1/2)*dq(3)*I5x*cos(q(5))^2*cos(q(3))+(1/2)*dq(3)*I5y*cos(q(5))^2*cos(q(3))+dq(5)*I5x*cos(q(4))*cos(q(3))-dq(5)*I5y*cos(q(4))*cos(q(3))+(9/4)*dq(3)*L4*L5*cos(q(4))*cos(q(5))*sin(q(3))*m5-(27/8)*dq(3)*L5^2*cos(q(4))*sin(q(5))*cos(q(5))*sin(q(3))*m5+(3/4)*dq(5)*L3*L5*cos(q(4))*sin(q(5))*cos(q(3))*m5+(3/4)*dq(5)*L4*L5*cos(q(4))*sin(q(5))*cos(q(3))*m5-(9/8)*L5^2*sin(q(5))*cos(q(5))*cos(q(3))*sin(q(4))*dq(4)*m5+(3/4)*L3*L5*cos(q(5))*cos(q(3))*sin(q(4))*dq(4)*m5+(3/4)*L4*L5*cos(q(5))*cos(q(3))*sin(q(4))*dq(4)*m5+(9/4)*dq(3)*L3*L5*cos(q(4))*cos(q(5))*sin(q(3))*m5;
Co(4,2)=0;
Co(4,3)=(1/4)*dq(1)*L3*L4*cos(q(4))*sin(q(3))*m4-(1/2)*dq(1)*I5y*cos(q(4))*sin(q(5))*cos(q(5))*sin(q(3))+(1/2)*dq(1)*I5x*cos(q(4))*sin(q(5))*cos(q(5))*sin(q(3))+(9/8)*L5^2*cos(q(4))*sin(q(5))*cos(q(5))*dq(4)*m5-(3/4)*L3*L5*cos(q(4))*cos(q(5))*dq(4)*m5-(3/4)*L4*L5*cos(q(4))*cos(q(5))*dq(4)*m5+(3/4)*L3*L5*sin(q(5))*sin(q(4))*dq(5)*m5+(3/4)*L4*L5*sin(q(5))*sin(q(4))*dq(5)*m5-I5y*cos(q(4))*sin(q(4))*dq(3)+I5z*cos(q(4))*sin(q(4))*dq(3)+(9/4)*dq(1)*L5^2*cos(q(4))^2*cos(q(5))^2*cos(q(3))*m5+(9/4)*L5^2*cos(q(4))*cos(q(5))^2*sin(q(4))*dq(3)*m5+(1/2)*dq(1)*I5x*cos(q(5))^2*cos(q(3))-(1/2)*dq(1)*I5y*cos(q(5))^2*cos(q(3))-(1/4)*L4^2*cos(q(4))*dq(4)*m4-2*I5x*cos(q(5))^2*sin(q(4))*dq(5)+2*I5y*cos(q(5))^2*sin(q(4))*dq(5)-(9/8)*L5^2*sin(q(4))*dq(5)*m5-(1/8)*dq(1)*m4*L4^2*cos(q(3))+(1/2)*dq(1)*I4x*cos(q(3))-(1/2)*dq(1)*I4z*cos(q(3))-(1/2)*dq(1)*I5z*cos(q(3))+(1/2)*I5z*sin(q(4))*dq(5)-dq(1)*I5x*cos(q(4))^2*cos(q(5))^2*cos(q(3))+dq(1)*I5y*cos(q(4))^2*cos(q(5))^2*cos(q(3))+(1/4)*dq(1)*L4^2*cos(q(4))^2*cos(q(3))*m4-I5x*cos(q(4))*cos(q(5))^2*sin(q(4))*dq(3)+I5y*cos(q(4))*cos(q(5))^2*sin(q(4))*dq(3)+(1/4)*L4^2*cos(q(4))*sin(q(4))*dq(3)*m4+(1/2)*dq(1)*I5y*cos(q(3))+I5x*sin(q(4))*dq(5)-I5y*sin(q(4))*dq(5)-dq(1)*I4x*cos(q(4))^2*cos(q(3))+dq(1)*I4z*cos(q(4))^2*cos(q(3))-dq(1)*I5y*cos(q(4))^2*cos(q(3))+dq(1)*I5z*cos(q(4))^2*cos(q(3))-I4x*cos(q(4))*sin(q(4))*dq(3)+I4z*cos(q(4))*sin(q(4))*dq(3)+(3/4)*dq(1)*L4*L5*cos(q(4))*cos(q(5))*sin(q(3))*m5-(9/8)*dq(1)*L5^2*cos(q(4))*sin(q(5))*cos(q(5))*sin(q(3))*m5+(3/4)*dq(1)*L3*L5*cos(q(4))*cos(q(5))*sin(q(3))*m5+(1/4)*dq(1)*L4^2*cos(q(4))*sin(q(3))*m4-(9/8)*dq(1)*L5^2*cos(q(5))^2*cos(q(3))*m5-(1/2)*I5x*cos(q(4))*sin(q(5))*cos(q(5))*dq(4)+(1/2)*I5y*cos(q(4))*sin(q(5))*cos(q(5))*dq(4)-(1/4)*L3*L4*cos(q(4))*dq(4)*m4+(9/2)*L5^2*cos(q(5))^2*sin(q(4))*dq(5)*m5;
Co(4,4)=-(9/2)*L5^2*sin(q(5))*cos(q(5))*dq(5)*m5+2*I5x*sin(q(5))*cos(q(5))*dq(5)-2*I5y*sin(q(5))*cos(q(5))*dq(5)+(9/8)*L5^2*sin(q(5))*cos(q(5))*cos(q(3))*sin(q(4))*dq(1)*m5-(3/4)*L3*L5*cos(q(5))*cos(q(3))*sin(q(4))*dq(1)*m5-(3/4)*L4*L5*cos(q(5))*cos(q(3))*sin(q(4))*dq(1)*m5-(1/2)*I5x*sin(q(5))*cos(q(5))*cos(q(3))*sin(q(4))*dq(1)+(1/2)*I5y*sin(q(5))*cos(q(5))*cos(q(3))*sin(q(4))*dq(1)-(3/4)*L2*L5*cos(q(5))*sin(q(4))*dq(1)*m5-(1/4)*L3*L4*cos(q(3))*sin(q(4))*dq(1)*m4-(1/4)*L4^2*cos(q(3))*sin(q(4))*dq(1)*m4-(1/4)*L2*L4*sin(q(4))*dq(1)*m4-(9/8)*L5^2*cos(q(4))*sin(q(5))*cos(q(5))*dq(3)*m5+(3/4)*L3*L5*cos(q(4))*cos(q(5))*dq(3)*m5+(3/4)*L4*L5*cos(q(4))*cos(q(5))*dq(3)*m5+(1/2)*I5x*cos(q(4))*sin(q(5))*cos(q(5))*dq(3)-(1/2)*I5y*cos(q(4))*sin(q(5))*cos(q(5))*dq(3)+(1/4)*L3*L4*cos(q(4))*dq(3)*m4+(1/4)*L4^2*cos(q(4))*dq(3)*m4;
Co(4,5)=-(3/4)*L3*L5*cos(q(4))*sin(q(5))*cos(q(3))*dq(1)*m5-(3/4)*L4*L5*cos(q(4))*sin(q(5))*cos(q(3))*dq(1)*m5-(3/4)*L2*L5*cos(q(4))*sin(q(5))*dq(1)*m5-(3/4)*L3*L5*sin(q(5))*sin(q(4))*dq(3)*m5-(3/4)*L4*L5*sin(q(5))*sin(q(4))*dq(3)*m5+(9/8)*L5^2*cos(q(4))*cos(q(3))*dq(1)*m5+(9/8)*L5^2*sin(q(4))*dq(3)*m5+(1/2)*I5z*cos(q(4))*cos(q(3))*dq(1)+(1/2)*I5z*sin(q(4))*dq(3);

Co(5,1)=(3/4)*L2*L5*cos(q(4))*sin(q(5))*dq(4)*m5+(3/4)*L2*L5*cos(q(5))*sin(q(4))*dq(5)*m5-dq(1)*I5x*cos(q(4))*cos(q(3))*sin(q(3))+dq(1)*I5y*cos(q(4))*cos(q(3))*sin(q(3))+dq(1)*I5x*cos(q(3))^2*cos(q(5))*sin(q(5))-dq(1)*I5y*cos(q(3))^2*cos(q(5))*sin(q(5))+(9/4)*dq(1)*L5^2*sin(q(5))*cos(q(5))*m5+dq(4)*I5x*cos(q(5))^2*cos(q(4))*cos(q(3))-dq(4)*I5y*cos(q(5))^2*cos(q(4))*cos(q(3))-dq(4)*I5x*sin(q(5))*cos(q(5))*sin(q(3))+dq(4)*I5y*sin(q(5))*cos(q(5))*sin(q(3))+I5x*cos(q(5))^2*sin(q(3))*sin(q(4))*dq(3)-I5y*cos(q(5))^2*sin(q(3))*sin(q(4))*dq(3)-(9/4)*L5^2*cos(q(4))*sin(q(5))*cos(q(5))*cos(q(3))*sin(q(4))*dq(3)*m5-(9/8)*L5^2*cos(q(4))*cos(q(3))*dq(4)*m5+(27/8)*L5^2*sin(q(3))*sin(q(4))*dq(3)*m5-(3/2)*dq(1)*m5*sin(q(3))*cos(q(4))*L5*sin(q(5))*L3*cos(q(3))-(3/2)*dq(1)*m5*sin(q(3))*cos(q(4))*L5*sin(q(5))*cos(q(3))*L4+(9/4)*dq(1)*m5*sin(q(3))*cos(q(4))*L5^2*cos(q(3))+dq(1)*I5x*cos(q(4))^2*cos(q(3))^2*cos(q(5))*sin(q(5))-dq(1)*I5y*cos(q(4))^2*cos(q(3))^2*cos(q(5))*sin(q(5))-(9/4)*dq(1)*L5^2*cos(q(5))*cos(q(3))^2*m5*sin(q(5))+2*dq(1)*I5x*cos(q(4))*cos(q(3))*sin(q(3))*cos(q(5))^2-2*dq(1)*I5y*cos(q(4))*cos(q(3))*sin(q(3))*cos(q(5))^2+(3/2)*dq(1)*m5*cos(q(3))^2*L5*cos(q(5))*L3+(3/2)*dq(1)*m5*cos(q(3))^2*L5*cos(q(5))*L4+(3/2)*dq(1)*m5*cos(q(3))*L5*cos(q(5))*L2-(9/4)*dq(4)*m5*L5^2*cos(q(5))^2*cos(q(4))*cos(q(3))+(9/4)*dq(4)*m5*L5^2*sin(q(5))*cos(q(5))*sin(q(3))-(9/4)*L5^2*cos(q(5))^2*sin(q(3))*sin(q(4))*dq(3)*m5-I5z*cos(q(4))*cos(q(3))*dq(4)+I5z*sin(q(3))*sin(q(4))*dq(3)-dq(1)*I5x*sin(q(5))*cos(q(5))+dq(1)*I5y*sin(q(5))*cos(q(5))-(1/2)*dq(4)*I5x*cos(q(4))*cos(q(3))+(1/2)*dq(4)*I5y*cos(q(4))*cos(q(3))-(1/2)*I5x*sin(q(3))*sin(q(4))*dq(3)+(1/2)*I5y*sin(q(3))*sin(q(4))*dq(3)-(9/4)*dq(1)*L5^2*cos(q(5))*cos(q(4))^2*cos(q(3))^2*m5*sin(q(5))-(9/2)*dq(1)*m5*sin(q(3))*cos(q(4))*L5^2*cos(q(5))^2*cos(q(3))-(3/2)*dq(1)*m5*L5*sin(q(5))*cos(q(4))*sin(q(3))*L2+I5x*cos(q(4))*sin(q(5))*cos(q(5))*cos(q(3))*sin(q(4))*dq(3)-I5y*cos(q(4))*sin(q(5))*cos(q(5))*cos(q(3))*sin(q(4))*dq(3)+(3/4)*L3*L5*cos(q(4))*sin(q(5))*cos(q(3))*dq(4)*m5-(9/4)*L3*L5*sin(q(5))*sin(q(3))*sin(q(4))*dq(3)*m5+(3/4)*L3*L5*cos(q(5))*cos(q(3))*sin(q(4))*dq(5)*m5+(3/4)*L4*L5*cos(q(4))*sin(q(5))*cos(q(3))*dq(4)*m5-(9/4)*L4*L5*sin(q(5))*sin(q(3))*sin(q(4))*dq(3)*m5+(3/4)*L4*L5*cos(q(5))*cos(q(3))*sin(q(4))*dq(5)*m5;
Co(5,2)=0;
Co(5,3)=-(9/8)*L5^2*sin(q(4))*dq(4)*m5+I5x*cos(q(5))^2*sin(q(3))*sin(q(4))*dq(1)-I5y*cos(q(5))^2*sin(q(3))*sin(q(4))*dq(1)-I5x*cos(q(4))^2*sin(q(5))*cos(q(5))*dq(3)+I5y*cos(q(4))^2*sin(q(5))*cos(q(5))*dq(3)-(9/4)*L5^2*sin(q(5))*cos(q(5))*dq(3)*m5+(3/2)*L3*L5*cos(q(5))*dq(3)*m5+(3/2)*L4*L5*cos(q(5))*dq(3)*m5-(9/4)*L5^2*cos(q(5))^2*sin(q(4))*dq(4)*m5-(9/4)*L5^2*cos(q(4))*sin(q(5))*cos(q(5))*cos(q(3))*sin(q(4))*dq(1)*m5-(9/4)*L5^2*cos(q(5))^2*sin(q(3))*sin(q(4))*dq(1)*m5+(9/4)*L5^2*cos(q(4))^2*sin(q(5))*cos(q(5))*dq(3)*m5-(3/4)*cos(q(4))*L5*cos(q(5))*m5*dq(5)*L4+(3/4)*L3*L5*sin(q(5))*sin(q(4))*dq(4)*m5-(3/4)*cos(q(4))*L5*cos(q(5))*m5*dq(5)*L3+(3/4)*L4*L5*sin(q(5))*sin(q(4))*dq(4)*m5+I5x*cos(q(4))*sin(q(5))*cos(q(5))*cos(q(3))*sin(q(4))*dq(1)-I5y*cos(q(4))*sin(q(5))*cos(q(5))*cos(q(3))*sin(q(4))*dq(1)-(1/2)*I5x*sin(q(4))*dq(4)+(1/2)*I5y*sin(q(4))*dq(4)+(9/8)*L5^2*sin(q(3))*sin(q(4))*dq(1)*m5-I5z*sin(q(4))*dq(4)-(1/2)*I5x*sin(q(3))*sin(q(4))*dq(1)+(1/2)*I5y*sin(q(3))*sin(q(4))*dq(1)+I5x*sin(q(5))*cos(q(5))*dq(3)-I5y*sin(q(5))*cos(q(5))*dq(3)+I5x*cos(q(5))^2*sin(q(4))*dq(4)-I5y*cos(q(5))^2*sin(q(4))*dq(4)-(3/4)*L3*L5*sin(q(5))*sin(q(3))*sin(q(4))*dq(1)*m5-(3/4)*L4*L5*sin(q(5))*sin(q(3))*sin(q(4))*dq(1)*m5;
Co(5,4)=-(9/4)*L5^2*cos(q(5))^2*sin(q(4))*dq(3)*m5-(3/4)*L3*L5*sin(q(5))*sin(q(4))*dq(3)*m5-(3/4)*L4*L5*sin(q(5))*sin(q(4))*dq(3)*m5+I5x*cos(q(5))^2*sin(q(4))*dq(3)-I5y*cos(q(5))^2*sin(q(4))*dq(3)+(9/8)*L5^2*sin(q(4))*dq(3)*m5-(1/2)*I5x*sin(q(4))*dq(3)+(1/2)*I5y*sin(q(4))*dq(3)+(9/4)*L5^2*sin(q(5))*cos(q(5))*dq(4)*m5-I5x*sin(q(5))*cos(q(5))*dq(4)+I5y*sin(q(5))*cos(q(5))*dq(4)-(9/4)*dq(1)*m5*L5^2*cos(q(5))^2*cos(q(4))*cos(q(3))+(9/8)*L5^2*cos(q(4))*cos(q(3))*dq(1)*m5-(3/4)*L3*L5*cos(q(4))*sin(q(5))*cos(q(3))*dq(1)*m5-(3/4)*L4*L5*cos(q(4))*sin(q(5))*cos(q(3))*dq(1)*m5+(9/4)*dq(1)*m5*L5^2*sin(q(5))*cos(q(5))*sin(q(3))+dq(1)*I5x*cos(q(5))^2*cos(q(4))*cos(q(3))-(1/2)*dq(1)*I5x*cos(q(4))*cos(q(3))-dq(1)*I5y*cos(q(5))^2*cos(q(4))*cos(q(3))+(1/2)*dq(1)*I5y*cos(q(4))*cos(q(3))-(3/4)*L2*L5*cos(q(4))*sin(q(5))*dq(1)*m5-dq(1)*I5x*sin(q(5))*cos(q(5))*sin(q(3))+dq(1)*I5y*sin(q(5))*cos(q(5))*sin(q(3));
Co(5,5)=-(3/4)*L5*cos(q(5))*m5*(L3*cos(q(3))*sin(q(4))*dq(1)+L4*cos(q(3))*sin(q(4))*dq(1)+L2*sin(q(4))*dq(1)-cos(q(4))*dq(3)*L3-cos(q(4))*dq(3)*L4);

% Ma tran the nang hap dan
G=zeros(5,1);
G(1,1)=0;
G(2,1)=5*m1;
G(3,1)=-15*m5*sin(q(3))*cos(q(4))*L5*cos(q(5))-5*m4*sin(q(3))*cos(q(4))*L4-15*m5*cos(q(3))*L5*sin(q(5))+15*m3*L3*cos(q(3))+10*m4*L3*cos(q(3))+10*m5*L3*cos(q(3))+10*m4*cos(q(3))*L4+10*m5*cos(q(3))*L4;
G(4,1)=-5*sin(q(4))*cos(q(3))*(3*L5*cos(q(5))*m5+m4*L4);
G(5,1)=-15*m5*L5*(cos(q(3))*cos(q(4))*sin(q(5))+sin(q(3))*cos(q(5)));
%chuyen doi luc sang luc suy rong
Fs=zeros(5,1);
Fs(1,1)=-150*L5*cos(q(5))*cos(q(4))*sin(q(3))*sin(q(1))-150*L5*cos(q(5))*sin(q(4))*cos(q(1))-150*sin(q(1))*cos(q(3))*L5*sin(q(5))+100*sin(q(1))*L3*cos(q(3))+100*sin(q(1))*cos(q(3))*L4+100*sin(q(1))*L2;
Fs(2,1)=0;
Fs(3,1)=50*cos(q(1))*(3*cos(q(3))*cos(q(4))*L5*cos(q(5))-3*sin(q(3))*L5*sin(q(5))+2*L3*sin(q(3))+2*sin(q(3))*L4)-150*sin(q(3))*cos(q(4))*L5*cos(q(5))-150*cos(q(3))*L5*sin(q(5))+100*L3*cos(q(3))+100*cos(q(3))*L4;
Fs(4,1)=-150*L5*cos(q(5))*(cos(q(1))*sin(q(3))*sin(q(4))+sin(q(1))*cos(q(4)))-150*cos(q(3))*sin(q(4))*L5*cos(q(5));
Fs(5,1)=150*L5*(-sin(q(5))*cos(q(4))*sin(q(3))*cos(q(1))+sin(q(5))*sin(q(4))*sin(q(1))+cos(q(1))*cos(q(3))*cos(q(5)))-150*L5*(cos(q(3))*cos(q(4))*sin(q(5))+sin(q(3))*cos(q(5)));
% Pt DLH
Tau=M*ddq + Co*dq + G + Fs;

== matlab function DLHnguoc_5DOF/q, dq, ddq ==
  data: t input; q output; dq output; ddq output
function [q,dq,ddq] = fcn(t)
a=0.4; b=0.7; c=0.8; d=1; e=1.2;
q1 = a*sin(t);
q2 = b*cos(t);
q3 = c*sin(t);
q4 = d*cos(t);
q5 = e*sin(t);

q=zeros(5,1);
q(1,1)=q1;
q(2,1)=q2;
q(3,1)=q3;
q(4,1)=q4;
q(5,1)=q5;

dq1=a*cos(t);
dq2=-b*sin(t);
dq3=c*cos(t);
dq4=-d*sin(t);
dq5=e*cos(t);

dq=zeros(5,1);
dq(1,1)=dq1;
dq(2,1)=dq2;
dq(3,1)=dq3;
dq(4,1)=dq4;
dq(5,1)=dq5;

ddq1=-a*sin(t);
ddq2=-b*cos(t);
ddq3=-c*sin(t);
ddq4=-d*cos(t);
ddq5=-e*sin(t);

ddq=zeros(5,1);
ddq(1,1)=ddq1;
ddq(2,1)=ddq2;
ddq(3,1)=ddq3;
ddq(4,1)=ddq4;
ddq(5,1)=ddq5;
